simulink model "AULA27"  (R2025b)
settings: Solver=VariableStepAuto  StartTime=0.0  StopTime=20  RelTol=1e-3

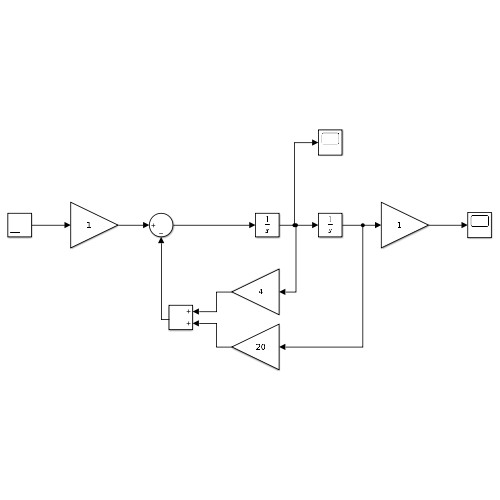
[thumbnail: Simulink's stored preview of the top-level diagram]
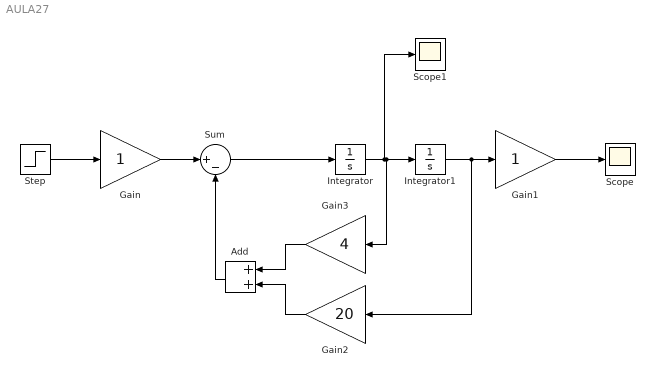
== system AULA27 ==
  Add : Sum
  Gain : Gain
  Gain1 : Gain
  Gain2 : Gain  Gain=20
  Gain3 : Gain  Gain=4
  Integrator : Integrator
  Integrator1 : Integrator
  Scope : Scope
      settings: ActiveDisplayYMinimum=-0.0074852654940674316  ActiveDisplayYMaximum=0.0673673894466069
  Scope1 : Scope
      settings: ActiveDisplayYMinimum=-0.045511169011037883  ActiveDisplayYMaximum=0.14702530916737078
  Step : Step  SampleTime=0
  Sum : Sum  Inputs=|+-
  wires:
  Step/1 -> Gain/1
  Gain/1 -> Sum/1
  Sum/1 -> Integrator/1
  Integrator/1 -> Scope1/1, Gain3/1, Integrator1/1
  Integrator1/1 -> Gain2/1, Gain1/1
  Gain1/1 -> Scope/1
  Gain3/1 -> Add/1
  Gain2/1 -> Add/2
  Add/1 -> Sum/2
